simulink model "A3_3"  (R2016b)
settings: Solver=VariableStepAuto  StartTime=0.0  StopTime=10.0  RelTol=1e-3
settings Model: Creator=jonathankirchman  LastModifiedBy=jonathankirchman

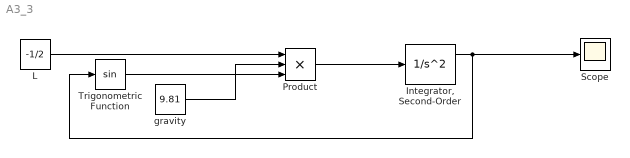
== system A3_3 ==
  "Integrator, Second-Order" : SecondOrderIntegrator  ICX=0.5
  L : Constant  Value=-1/2
  Product : Product  Inputs=3
  Scope : Scope
  Trigonometric Function : Trigonometry
  gravity : Constant  Value=9.81
  wires:
  L/1 -> Product/1
  gravity/1 -> Product/2
  Trigonometric Function/1 -> Product/3
  Product/1 -> "Integrator, Second-Order"/1
  "Integrator, Second-Order"/1 -> Trigonometric Function/1, Scope/1
